simulink model "top_level"  (R2019b)
settings: Solver=VariableStepAuto  StartTime=0.0  StopTime=10.0  RelTol=1e-3
settings Model: Creator=enrique.babio  LastModifiedBy=enrique.babio

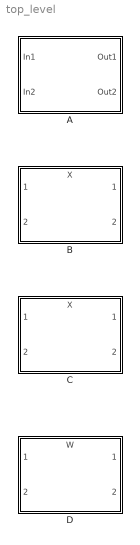
== system top_level ==
  A : Subsystem
  B : ModelReference  ModelNameDialog=X  SimulationMode=Normal  ModelReferenceVersion=1.3
  C : ModelReference  ModelNameDialog=X  SimulationMode=Normal  ModelReferenceVersion=1.3
  D : ModelReference  ModelNameDialog=W  SimulationMode=Normal  ModelReferenceVersion=1.3

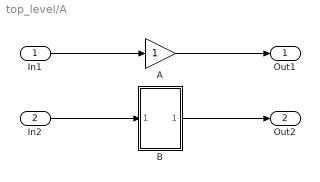
== system top_level/A ==
  In1 : Inport
  In2 : Inport  Port=2
  A : Gain
  B : Subsystem  ReferencedSubsystem=Y
  Out1 : Outport
  Out2 : Outport  Port=2
  wires:
  In1/1 -> A/1
  A/1 -> Out1/1
  In2/1 -> B/1
  B/1 -> Out2/1
